simulink library "autolibshared"  (R2019b)
settings: Solver=ode45  StartTime=0.0  StopTime=10.0  RelTol=1e-3  EnableMultiTasking=on
undefined symbols (not defined in the file or in its folder): AccelCycle, aMode, DriveCycle, GearCycle, psi, x_o
libraries: autolibsharedcommon x20, $bdroot x7, autolibutils x2, autolibpowerinfoutils x1
(part 4 of 4)

== system autolibshared/Longitudinal Wheel/Wheel Module/Clutch/detectLockup/Friction Mode Logic ==
  note: Clutch Friction Mode Logic
  Tout : Inport
  Tfmaxs : Inport  Port=2
  locked_wout : Inport  Port=3
  Break Apart Detection : Subsystem
  Lockup Detection : Subsystem
  Lockup FSM : Subsystem
  Requisite Friction : Subsystem
  locked : Outport  InitialOutput=0  VectorParamsAs1DForOutWhenUnconnected=off
  wires:
  Tfmaxs/1 -> Break Apart Detection/1(Tfmaxs), Lockup Detection/2(Tfmaxs)
  Requisite Friction/1(Tf) -> Break Apart Detection/2(Tf)
  Break Apart Detection/1(unlock) -> Lockup FSM/2(unlock)
  Lockup Detection/1(lock) -> Lockup FSM/1(lock)
  Lockup FSM/1(locked) -> locked/1
  locked_wout/1 -> Requisite Friction/2(locked_w)
  Tout/1 -> Requisite Friction/1(Tout), Lockup Detection/1(Tout)

== system autolibshared/Longitudinal Wheel/Wheel Module/Clutch/detectSlip/Break Apart Detection ==
  Tfmaxs : Inport
  Tf : Inport  Port=2
  Abs : Abs  SaturateOnIntegerOverflow=on
  Relational Operator : RelationalOperator  OutDataTypeStr=boolean  RndMeth=Nearest  InputSameDT=on
  unlock : Outport  InitialOutput=0  VectorParamsAs1DForOutWhenUnconnected=off
  wires:
  Tf/1 -> Abs/1
  Relational Operator/1 -> unlock/1
  Abs/1 -> Relational Operator/1
  Tfmaxs/1 -> Relational Operator/2

== system autolibshared/Vehicle Body 3DOF Single Track/Cy/Cy table dual/For Each Subsystem ==
  alpha_f : Inport  Partition=on  PartitionDimension=1  PartitionWidth=1  PartitionOffset=0
  alpha_r : Inport  Port=2  Partition=on  PartitionDimension=1  PartitionWidth=1  PartitionOffset=0
  Cy_f(alpha_f) : Lookup_n-D  NumberOfTableDimensions=1  BreakpointsForDimension1=alpha_f_brk  Table=Cy_f_data  ExtrapMethod=Clip  InternalRulePriority=Speed  RndMeth=Simplest  InputSameDT=on
  Cy_r(alpha_r) : Lookup_n-D  NumberOfTableDimensions=1  BreakpointsForDimension1=alpha_r_brk  Table=Cy_r_data  ExtrapMethod=Clip  InternalRulePriority=Speed  RndMeth=Simplest  InputSameDT=on
  For Each : ForEach  DisableCoverage=on
  Cy_f : Outport  ConcatenationDimension=1  VectorParamsAs1DForOutWhenUnconnected=off
  Cy_r : Outport  Port=2  ConcatenationDimension=1  VectorParamsAs1DForOutWhenUnconnected=off
  wires:
  alpha_f/1 -> Cy_f(alpha_f)/1
  Cy_f(alpha_f)/1 -> Cy_f/1
  alpha_r/1 -> Cy_r(alpha_r)/1
  Cy_r(alpha_r)/1 -> Cy_r/1

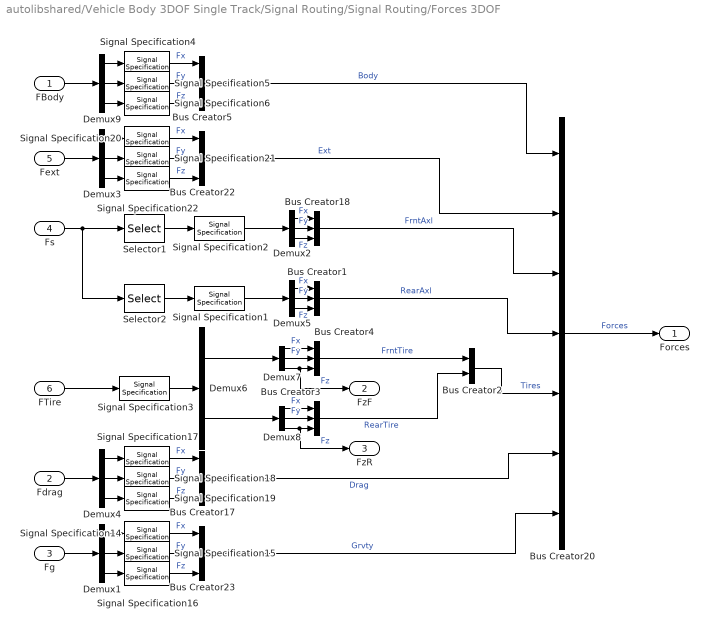
== system autolibshared/Vehicle Body 3DOF Single Track/Signal Routing/Signal Routing/Forces 3DOF ==
  FBody : Inport
  Fdrag : Inport  Port=2
  Fg : Inport  Port=3
  Fs : Inport  Port=4  Unit=N
  Fext : Inport  Port=5
  FTire : Inport  Port=6
  Bus Creator{1,3..5,17..18,22..23} (8 alike) : BusCreator  Inputs=3
  Bus Creator2 : BusCreator  Inputs=2
  Bus Creator20 : BusCreator  Inputs=7
  Demux{1..5,7..9} (8 alike) : Demux  Outputs=3
  Demux6 : Demux  Outputs=[3,3]
  Selector1 : Selector  IndexOptions=Index vector (dialog)  Indices=[1:3]  OutputSizes=1
  Selector2 : Selector  IndexOptions=Index vector (dialog)  Indices=[4:6]  OutputSizes=1
  Signal Specification{1..6,14..22} (15 alike) : SignalSpecification  Unit=N
  Forces : Outport  VectorParamsAs1DForOutWhenUnconnected=off
  FzF : Outport  Port=2  VectorParamsAs1DForOutWhenUnconnected=off
  FzR : Outport  Port=3  VectorParamsAs1DForOutWhenUnconnected=off
  wires:
  Signal Specification5/1 -> Bus Creator5/2  "Fy"
  Signal Specification4/1 -> Bus Creator5/1  "Fx"
  Signal Specification6/1 -> Bus Creator5/3  "Fz"
  FBody/1 -> Demux9/1
  Demux9/1 -> Signal Specification4/1
  Demux9/2 -> Signal Specification5/1
  Demux9/3 -> Signal Specification6/1
  Bus Creator5/1 -> Bus Creator20/1  "Body"
  Bus Creator17/1 -> Bus Creator20/6  "Drag"
  Bus Creator2/1 -> Bus Creator20/5  "Tires"
  Demux6/2 -> Demux8/1
  Demux6/1 -> Demux7/1
  Signal Specification3/1 -> Demux6/1
  FTire/1 -> Signal Specification3/1
  Selector2/1 -> Signal Specification1/1
  Signal Specification2/1 -> Demux2/1
  Signal Specification1/1 -> Demux5/1
  Fs/1 -> Selector2/1, Selector1/1
  Selector1/1 -> Signal Specification2/1
  Demux5/1 -> Bus Creator1/1  "Fx"
  Bus Creator4/1 -> Bus Creator2/1  "FrntTire"
  Bus Creator3/1 -> Bus Creator2/2  "RearTire"
  Demux7/1 -> Bus Creator4/1  "Fx"
  Demux7/2 -> Bus Creator4/2  "Fy"
  Demux7/3 -> Bus Creator4/3, FzF/1  "Fz"
  Demux8/3 -> Bus Creator3/3, FzR/1  "Fz"
  Demux8/2 -> Bus Creator3/2  "Fy"
  Demux8/1 -> Bus Creator3/1  "Fx"
  Demux5/2 -> Bus Creator1/2  "Fy"
  Demux5/3 -> Bus Creator1/3  "Fz"
  Demux2/3 -> Bus Creator18/3  "Fz"
  Demux2/2 -> Bus Creator18/2  "Fy"
  Demux2/1 -> Bus Creator18/1  "Fx"
  Bus Creator1/1 -> Bus Creator20/4  "RearAxl"
  Bus Creator18/1 -> Bus Creator20/3  "FrntAxl"
  Fdrag/1 -> Demux4/1
  Demux4/3 -> Signal Specification19/1
  Demux4/2 -> Signal Specification18/1
  Demux4/1 -> Signal Specification17/1
  Demux3/3 -> Signal Specification22/1
  Demux3/2 -> Signal Specification21/1
  Demux3/1 -> Signal Specification20/1
  Fext/1 -> Demux3/1
  Bus Creator22/1 -> Bus Creator20/2  "Ext"
  Signal Specification22/1 -> Bus Creator22/3  "Fz"
  Signal Specification20/1 -> Bus Creator22/1  "Fx"
  Signal Specification15/1 -> Bus Creator23/2  "Fy"
  Signal Specification21/1 -> Bus Creator22/2  "Fy"
  Signal Specification18/1 -> Bus Creator17/2  "Fy"
  Signal Specification17/1 -> Bus Creator17/1  "Fx"
  Signal Specification14/1 -> Bus Creator23/1  "Fx"
  Signal Specification19/1 -> Bus Creator17/3  "Fz"
  Signal Specification16/1 -> Bus Creator23/3  "Fz"
  Bus Creator20/1 -> Forces/1  "Forces"
  Bus Creator23/1 -> Bus Creator20/7  "Grvty"
  Demux1/2 -> Signal Specification15/1
  Demux1/3 -> Signal Specification16/1
  Fg/1 -> Demux1/1
  Demux1/1 -> Signal Specification14/1

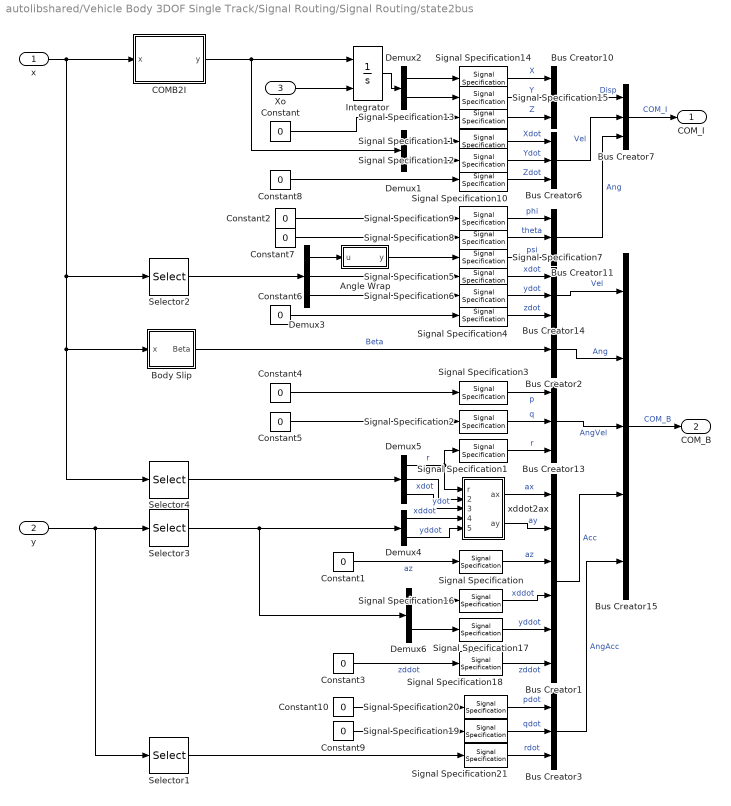
== system autolibshared/Vehicle Body 3DOF Single Track/Signal Routing/Signal Routing/state2bus ==
  x : Inport
  y : Inport  Port=2
  Xo : Inport  Port=3
  Angle Wrap : Subsystem  VariantControlMode=Label  Variant=on  VariantControl=Variant1  LabelModeActiveChoice=None
  Body Slip : Subsystem
  Bus Creator1 : BusCreator  Inputs=6
  Bus Creator{3,6..7,10..11,13..14} (7 alike) : BusCreator  Inputs=3
  Bus Creator15 : BusCreator  Inputs=5
  Bus Creator2 : BusCreator  Inputs=1
  COMB2I : MATLAB Function  TreatAsAtomicUnit=on
  Constant{,1..10} (11 alike) : Constant  Value=0
  Demux{1..2,4,6} (4 alike) : Demux  Outputs=2
  Demux3 : Demux  Outputs=3
  Demux5 : Demux  Outputs=3
  Integrator : Integrator  InitialConditionSource=external
  Selector1 : Selector  IndexOptions=Index vector (dialog)  Indices=[3]  OutputSizes=1
  Selector2 : Selector  IndexOptions=Index vector (dialog)  Indices=[3,1,2]  OutputSizes=1
  Selector3 : Selector  IndexOptions=Index vector (dialog)  Indices=[1,2]  OutputSizes=1
  Selector4 : Selector  IndexOptions=Index vector (dialog)  Indices=[4,1,2]  OutputSizes=1
  Signal Specification : SignalSpecification  Unit=gn
  Signal Specification1 : SignalSpecification  Unit=rad/s
  Signal Specification{4..6,10..12} (6 alike) : SignalSpecification  Unit=m/s
  Signal Specification13 : SignalSpecification  Unit=m
  Signal Specification14 : SignalSpecification  Unit=m
  Signal Specification15 : SignalSpecification  Unit=m
  Signal Specification16 : SignalSpecification  Unit=m/s^2
  Signal Specification17 : SignalSpecification  Unit=m/s^2
  Signal Specification18 : SignalSpecification  Unit=m/s^2
  Signal Specification19 : SignalSpecification  Unit=rad/s^2
  Signal Specification2 : SignalSpecification  Unit=rad/s
  Signal Specification20 : SignalSpecification  Unit=rad/s^2
  Signal Specification21 : SignalSpecification  Unit=rad/s^2
  Signal Specification3 : SignalSpecification  Unit=rad/s
  Signal Specification7 : SignalSpecification  Unit=rad
  Signal Specification8 : SignalSpecification  Unit=rad
  Signal Specification9 : SignalSpecification  Unit=rad
  xddot2ax : Subsystem
  COM_I : Outport  VectorParamsAs1DForOutWhenUnconnected=off
  COM_B : Outport  Port=2  VectorParamsAs1DForOutWhenUnconnected=off
  wires:
  Demux2/1 -> Signal Specification14/1
  Demux2/2 -> Signal Specification15/1
  Constant/1 -> Signal Specification13/1
  Demux1/1 -> Signal Specification11/1
  Demux1/2 -> Signal Specification12/1
  Constant2/1 -> Signal Specification9/1
  Constant7/1 -> Signal Specification8/1
  Demux3/1 -> Angle Wrap/1("u ")
  Demux3/3 -> Signal Specification6/1
  Demux3/2 -> Signal Specification5/1
  Constant6/1 -> Signal Specification4/1
  Constant4/1 -> Signal Specification3/1
  Constant5/1 -> Signal Specification2/1
  Signal Specification1/1 -> Bus Creator13/3  "r"
  xddot2ax/2(ay) -> Bus Creator1/2  "ay"
  xddot2ax/1(ax) -> Bus Creator1/1  "ax"
  Demux4/2 -> xddot2ax/5(yddot)  "yddot"
  Demux4/1 -> xddot2ax/4(xddot)  "xddot"
  Demux5/3 -> xddot2ax/3(ydot)  "ydot"
  Demux5/2 -> xddot2ax/2(xdot)  "xdot"
  Selector4/1 -> Demux5/1
  Demux5/1 -> xddot2ax/1(r), Signal Specification1/1  "r"
  x/1 -> Selector4/1, Body Slip/1(x), Selector2/1, COMB2I/1(x)
  Signal Specification10/1 -> Bus Creator6/3  "Zdot"
  Signal Specification4/1 -> Bus Creator14/3  "zdot"
  Signal Specification11/1 -> Bus Creator6/1  "Xdot"
  Signal Specification15/1 -> Bus Creator10/2  "Y"
  Bus Creator13/1 -> Bus Creator15/3  "AngVel"
  Signal Specification13/1 -> Bus Creator10/3  "Z"
  Signal Specification14/1 -> Bus Creator10/1  "X"
  Signal Specification9/1 -> Bus Creator11/1  "phi"
  Bus Creator7/1 -> COM_I/1  "COM_I"
  Signal Specification3/1 -> Bus Creator13/1  "p"
  Bus Creator14/1 -> Bus Creator15/1  "Vel"
  Bus Creator6/1 -> Bus Creator7/2  "Vel"
  Bus Creator10/1 -> Bus Creator7/1  "Disp"
  Signal Specification8/1 -> Bus Creator11/2  "theta"
  Selector2/1 -> Demux3/1
  Signal Specification12/1 -> Bus Creator6/2  "Ydot"
  Signal Specification2/1 -> Bus Creator13/2  "q"
  Bus Creator15/1 -> COM_B/1  "COM_B"
  Signal Specification5/1 -> Bus Creator14/1  "xdot"
  Bus Creator11/1 -> Bus Creator7/3  "Ang"
  Signal Specification6/1 -> Bus Creator14/2  "ydot"
  Integrator/1 -> Demux2/1
  COMB2I/1(y) -> Integrator/1, Demux1/1
  Signal Specification7/1 -> Bus Creator11/3  "psi"
  Signal Specification/1 -> Bus Creator1/3  "az"
  y/1 -> Selector1/1, Selector3/1
  Selector3/1 -> Demux4/1, Demux6/1
  Constant3/1 -> Signal Specification18/1  "zddot"
  Signal Specification18/1 -> Bus Creator1/6  "zddot"
  Signal Specification17/1 -> Bus Creator1/5  "yddot"
  Signal Specification16/1 -> Bus Creator1/4  "xddot"
  Constant1/1 -> Signal Specification/1  "az"
  Demux6/1 -> Signal Specification16/1
  Demux6/2 -> Signal Specification17/1
  Constant8/1 -> Signal Specification10/1
  Bus Creator1/1 -> Bus Creator15/4  "Acc"
  Bus Creator2/1 -> Bus Creator15/2  "Ang"
  Body Slip/1(Beta) -> Bus Creator2/1  "Beta"
  Xo/1 -> Integrator/2
  Signal Specification21/1 -> Bus Creator3/3  "rdot"
  Signal Specification19/1 -> Bus Creator3/2  "qdot"
  Signal Specification20/1 -> Bus Creator3/1  "pdot"
  Bus Creator3/1 -> Bus Creator15/5  "AngAcc"
  Constant9/1 -> Signal Specification19/1
  Constant10/1 -> Signal Specification20/1
  Selector1/1 -> Signal Specification21/1
  Angle Wrap/1(" y") -> Signal Specification7/1

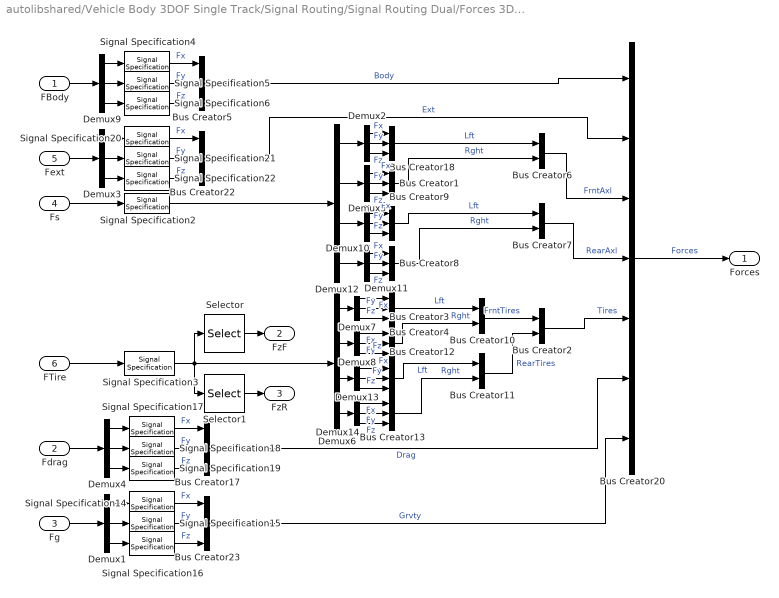
== system autolibshared/Vehicle Body 3DOF Single Track/Signal Routing/Signal Routing Dual/Forces 3DOF ==
  FBody : Inport
  Fdrag : Inport  Port=2
  Fg : Inport  Port=3
  Fs : Inport  Port=4  Unit=N
  Fext : Inport  Port=5
  FTire : Inport  Port=6
  Bus Creator{1,3..5,8..9,12..13,17..18,22..23} (12 alike) : BusCreator  Inputs=3
  Bus Creator{2,6..7,10..11} (5 alike) : BusCreator  Inputs=2
  Bus Creator20 : BusCreator  Inputs=7
  Demux{1..5,7..11,13..14} (12 alike) : Demux  Outputs=3
  Demux12 : Demux  Outputs=[3,3,3,3]
  Demux6 : Demux  Outputs=[3,3,3,3]
  Selector : Selector  InputPortWidth=12  IndexOptions=Index vector (dialog)  Indices=[3,6]  OutputSizes=1
  Selector1 : Selector  InputPortWidth=12  IndexOptions=Index vector (dialog)  Indices=[9,12]  OutputSizes=1
  Signal Specification{2..6,14..22} (14 alike) : SignalSpecification  Unit=N
  Forces : Outport  VectorParamsAs1DForOutWhenUnconnected=off
  FzF : Outport  Port=2  VectorParamsAs1DForOutWhenUnconnected=off
  FzR : Outport  Port=3  VectorParamsAs1DForOutWhenUnconnected=off
  wires:
  Selector1/1 -> FzR/1
  Selector/1 -> FzF/1
  Demux13/3 -> Bus Creator12/3  "Fz"
  Bus Creator13/1 -> Bus Creator11/2  "Rght"
  Demux14/1 -> Bus Creator13/1  "Fx"
  Demux14/2 -> Bus Creator13/2  "Fy"
  Demux14/3 -> Bus Creator13/3  "Fz"
  Demux6/4 -> Demux14/1
  Demux6/3 -> Demux13/1
  Demux13/2 -> Bus Creator12/2  "Fy"
  Demux13/1 -> Bus Creator12/1  "Fx"
  Signal Specification2/1 -> Demux12/1
  Bus Creator12/1 -> Bus Creator11/1  "Lft"
  Bus Creator3/1 -> Bus Creator10/2  "Rght"
  Bus Creator4/1 -> Bus Creator10/1  "Lft"
  Demux12/3 -> Demux10/1
  Demux12/4 -> Demux11/1
  Demux11/1 -> Bus Creator8/1  "Fx"
  Demux11/2 -> Bus Creator8/2  "Fy"
  Demux11/3 -> Bus Creator8/3  "Fz"
  Demux10/3 -> Bus Creator9/3  "Fz"
  Demux10/2 -> Bus Creator9/2  "Fy"
  Demux10/1 -> Bus Creator9/1  "Fx"
  Bus Creator9/1 -> Bus Creator7/1  "Lft"
  Bus Creator8/1 -> Bus Creator7/2  "Rght"
  Bus Creator1/1 -> Bus Creator6/2  "Rght"
  Bus Creator18/1 -> Bus Creator6/1  "Lft"
  Demux1/1 -> Signal Specification14/1
  Fg/1 -> Demux1/1
  Demux1/3 -> Signal Specification16/1
  Demux1/2 -> Signal Specification15/1
  Bus Creator23/1 -> Bus Creator20/7  "Grvty"
  Bus Creator20/1 -> Forces/1  "Forces"
  Signal Specification16/1 -> Bus Creator23/3  "Fz"
  Signal Specification19/1 -> Bus Creator17/3  "Fz"
  Signal Specification14/1 -> Bus Creator23/1  "Fx"
  Signal Specification17/1 -> Bus Creator17/1  "Fx"
  Signal Specification18/1 -> Bus Creator17/2  "Fy"
  Signal Specification21/1 -> Bus Creator22/2  "Fy"
  Signal Specification15/1 -> Bus Creator23/2  "Fy"
  Signal Specification20/1 -> Bus Creator22/1  "Fx"
  Signal Specification22/1 -> Bus Creator22/3  "Fz"
  Bus Creator22/1 -> Bus Creator20/2  "Ext"
  Fext/1 -> Demux3/1
  Demux3/1 -> Signal Specification20/1
  Demux3/2 -> Signal Specification21/1
  Demux3/3 -> Signal Specification22/1
  Demux4/1 -> Signal Specification17/1
  Demux4/2 -> Signal Specification18/1
  Demux4/3 -> Signal Specification19/1
  Fdrag/1 -> Demux4/1
  Bus Creator6/1 -> Bus Creator20/3  "FrntAxl"
  Bus Creator7/1 -> Bus Creator20/4  "RearAxl"
  Demux2/1 -> Bus Creator18/1  "Fx"
  Demux2/2 -> Bus Creator18/2  "Fy"
  Demux2/3 -> Bus Creator18/3  "Fz"
  Demux5/3 -> Bus Creator1/3  "Fz"
  Demux5/2 -> Bus Creator1/2  "Fy"
  Demux8/1 -> Bus Creator3/1  "Fx"
  Demux8/2 -> Bus Creator3/2  "Fy"
  Demux8/3 -> Bus Creator3/3  "Fz"
  Demux7/3 -> Bus Creator4/3  "Fz"
  Demux7/2 -> Bus Creator4/2  "Fy"
  Demux7/1 -> Bus Creator4/1  "Fx"
  Bus Creator11/1 -> Bus Creator2/2  "RearTires"
  Bus Creator10/1 -> Bus Creator2/1  "FrntTires"
  Demux5/1 -> Bus Creator1/1  "Fx"
  Fs/1 -> Signal Specification2/1
  Demux12/2 -> Demux5/1
  Demux12/1 -> Demux2/1
  FTire/1 -> Signal Specification3/1
  Signal Specification3/1 -> Demux6/1, Selector/1, Selector1/1
  Demux6/1 -> Demux7/1
  Demux6/2 -> Demux8/1
  Bus Creator2/1 -> Bus Creator20/5  "Tires"
  Bus Creator17/1 -> Bus Creator20/6  "Drag"
  Bus Creator5/1 -> Bus Creator20/1  "Body"
  Demux9/3 -> Signal Specification6/1
  Demux9/2 -> Signal Specification5/1
  Demux9/1 -> Signal Specification4/1
  FBody/1 -> Demux9/1
  Signal Specification6/1 -> Bus Creator5/3  "Fz"
  Signal Specification4/1 -> Bus Creator5/1  "Fx"
  Signal Specification5/1 -> Bus Creator5/2  "Fy"

== system autolibshared/Vehicle Body 3DOF Single Track/Signal Routing/Signal Routing Dual/Lateral 3DOF ==
  InertCg : Inport
  BdyFrmCg : Inport  Port=2
  Forces : Inport  Port=3
  Power : Inport  Port=4
  Moments : Inport  Port=5
  WhlAngF : Inport  Port=6
  WhlAngR : Inport  Port=7
  Bus Creator1 : BusCreator  Inputs=7
  Bus Creator2 : BusCreator  Inputs=4
  Bus Creator{3..4,7..8} (4 alike) : BusCreator  Inputs=2
  Bus Creator5 : BusCreator  Inputs=3
  Bus Creator6 : BusCreator  Inputs=3
  Bus Selector : BusSelector  OutputSignals=Pwr,PwrInfo
  Demux : Demux  Outputs=2
  Demux1 : Demux  Outputs=2
  Hard Point Coordinate Transform Front Left : Subsystem
  Hard Point Coordinate Transform Front Right : Subsystem
  Hard Point Coordinate Transform Geometric : Subsystem
  Hard Point Coordinate Transform Rear Left : Subsystem
  Hard Point Coordinate Transform Rear Right : Subsystem
  InertFrm : Outport  VectorParamsAs1DForOutWhenUnconnected=off
  BdyFrm : Outport  Port=2  VectorParamsAs1DForOutWhenUnconnected=off
  PwrInfo : Outport  Port=3  VectorParamsAs1DForOutWhenUnconnected=off
  wires:
  Bus Creator6/1 -> Bus Creator1/5  "RearAxl"
  Hard Point Coordinate Transform Front Left/2(Body) -> Bus Creator5/1  "Lft"
  Hard Point Coordinate Transform Front Right/2(Body) -> Bus Creator5/2  "Rght"
  Hard Point Coordinate Transform Rear Left/2(Body) -> Bus Creator6/1  "Lft"
  Hard Point Coordinate Transform Rear Right/2(Body) -> Bus Creator6/2  "Rght"
  Hard Point Coordinate Transform Rear Right/1(Inert) -> Bus Creator4/2  "Rght"
  Hard Point Coordinate Transform Rear Left/1(Inert) -> Bus Creator4/1  "Lft"
  Hard Point Coordinate Transform Front Right/1(Inert) -> Bus Creator3/2  "Rght"
  Hard Point Coordinate Transform Front Left/1(Inert) -> Bus Creator3/1  "Lft"
  Moments/1 -> Bus Creator1/3  "Moments"
  Bus Creator5/1 -> Bus Creator1/4  "FrntAxl"
  InertCg/1 -> Hard Point Coordinate Transform Front Left/1(InertFrmCg), Bus Creator2/1, Hard Point Coordinate Transform Front Right/1(InertFrmCg), Hard Point Coordinate Transform Geometric/1(InertFrmCg), Hard Point Coordinate Transform Rear Right/1(InertFrmCg), Hard Point Coordinate Transform Rear Left/1(InertFrmCg)  "Cg"
  Bus Creator4/1 -> Bus Creator2/3  "RearAxl"
  Bus Creator2/1 -> InertFrm/1  "InertFrm"
  Bus Creator1/1 -> BdyFrm/1  "BdyFrm"
  Bus Creator3/1 -> Bus Creator2/2  "FrntAxl"
  BdyFrmCg/1 -> Hard Point Coordinate Transform Geometric/2(BdyFrmCg), Bus Creator1/1, Hard Point Coordinate Transform Rear Right/2(BdyFrmCg), Hard Point Coordinate Transform Rear Left/2(BdyFrmCg), Hard Point Coordinate Transform Front Right/2(BdyFrmCg), Hard Point Coordinate Transform Front Left/2(BdyFrmCg)  "Cg"
  Forces/1 -> Bus Creator1/2  "Forces"
  Hard Point Coordinate Transform Geometric/2(Body) -> Bus Creator1/7  "Geom"
  Hard Point Coordinate Transform Geometric/1(Inert) -> Bus Creator2/4  "Geom"
  WhlAngF/1 -> Demux/1  "WhlAngF"
  WhlAngR/1 -> Demux1/1  "WhlAngR"
  Bus Creator7/1 -> Bus Creator6/3  "Steer"
  Bus Creator8/1 -> Bus Creator5/3  "Steer"
  Demux/1 -> Bus Creator8/1  "WhlAngFL"
  Demux/2 -> Bus Creator8/2  "WhlAngFR"
  Demux1/1 -> Bus Creator7/1  "WhlAngRL"
  Demux1/2 -> Bus Creator7/2  "WhlAngRR"
  Bus Selector/2 -> PwrInfo/1  "<PwrInfo>"
  Bus Selector/1 -> Bus Creator1/6  "<Pwr>"
  Power/1 -> Bus Selector/1  "Pwr"

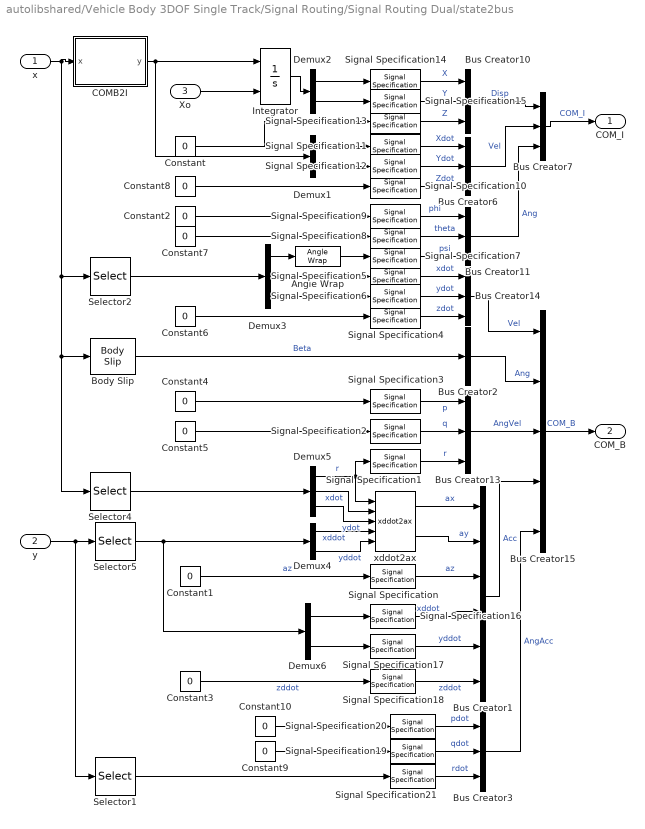
== system autolibshared/Vehicle Body 3DOF Single Track/Signal Routing/Signal Routing Dual/state2bus ==
  x : Inport
  y : Inport  Port=2
  Xo : Inport  Port=3
  Angle Wrap : $bdroot/Vehicle Body 3DOF Single Track/Signal Routing/Signal Routing/state2bus/Angle Wrap  SystemSampleTime=-1  VariantControl=Variant1  LabelModeActiveChoice=None  Latency=0  AutoFrameSizeCalculation=off
  Body Slip : $bdroot/Vehicle Body 3DOF Single Track/Signal Routing/Signal Routing/state2bus/Body Slip  SystemSampleTime=-1  Latency=0  AutoFrameSizeCalculation=off
  Bus Creator1 : BusCreator  Inputs=6
  Bus Creator{3,6..7,10..11,13..14} (7 alike) : BusCreator  Inputs=3
  Bus Creator15 : BusCreator  Inputs=5
  Bus Creator2 : BusCreator  Inputs=1
  COMB2I : MATLAB Function  TreatAsAtomicUnit=on
  Constant{,1..10} (11 alike) : Constant  Value=0
  Demux{1..2,4,6} (4 alike) : Demux  Outputs=2
  Demux3 : Demux  Outputs=3
  Demux5 : Demux  Outputs=3
  Integrator : Integrator  InitialConditionSource=external
  Selector1 : Selector  IndexOptions=Index vector (dialog)  Indices=[3]  OutputSizes=1
  Selector2 : Selector  IndexOptions=Index vector (dialog)  Indices=[3,1,2]  OutputSizes=1
  Selector4 : Selector  IndexOptions=Index vector (dialog)  Indices=[4,1,2]  OutputSizes=1
  Selector5 : Selector  IndexOptions=Index vector (dialog)  Indices=[1,2]  OutputSizes=1
  Signal Specification : SignalSpecification  Unit=gn
  Signal Specification1 : SignalSpecification  Unit=rad/s
  Signal Specification{4..6,10..12} (6 alike) : SignalSpecification  Unit=m/s
  Signal Specification13 : SignalSpecification  Unit=m
  Signal Specification14 : SignalSpecification  Unit=m
  Signal Specification15 : SignalSpecification  Unit=m
  Signal Specification16 : SignalSpecification  Unit=m/s^2
  Signal Specification17 : SignalSpecification  Unit=m/s^2
  Signal Specification18 : SignalSpecification  Unit=m/s^2
  Signal Specification19 : SignalSpecification  Unit=rad/s^2
  Signal Specification2 : SignalSpecification  Unit=rad/s
  Signal Specification20 : SignalSpecification  Unit=rad/s^2
  Signal Specification21 : SignalSpecification  Unit=rad/s^2
  Signal Specification3 : SignalSpecification  Unit=rad/s
  Signal Specification7 : SignalSpecification  Unit=rad
  Signal Specification8 : SignalSpecification  Unit=rad
  Signal Specification9 : SignalSpecification  Unit=rad
  xddot2ax : $bdroot/Vehicle Body 3DOF Single Track/Signal Routing/Signal Routing/state2bus/xddot2ax  SystemSampleTime=-1  Latency=0  AutoFrameSizeCalculation=off
  COM_I : Outport  VectorParamsAs1DForOutWhenUnconnected=off
  COM_B : Outport  Port=2  VectorParamsAs1DForOutWhenUnconnected=off
  wires:
  Signal Specification7/1 -> Bus Creator11/3  "psi"
  COMB2I/1(y) -> Demux1/1, Integrator/1
  Integrator/1 -> Demux2/1
  Signal Specification6/1 -> Bus Creator14/2  "ydot"
  Bus Creator11/1 -> Bus Creator7/3  "Ang"
  Signal Specification5/1 -> Bus Creator14/1  "xdot"
  Bus Creator15/1 -> COM_B/1  "COM_B"
  Signal Specification2/1 -> Bus Creator13/2  "q"
  Signal Specification12/1 -> Bus Creator6/2  "Ydot"
  Selector2/1 -> Demux3/1
  Signal Specification8/1 -> Bus Creator11/2  "theta"
  Bus Creator10/1 -> Bus Creator7/1  "Disp"
  Bus Creator6/1 -> Bus Creator7/2  "Vel"
  Bus Creator14/1 -> Bus Creator15/1  "Vel"
  Signal Specification3/1 -> Bus Creator13/1  "p"
  Bus Creator7/1 -> COM_I/1  "COM_I"
  Signal Specification9/1 -> Bus Creator11/1  "phi"
  Signal Specification14/1 -> Bus Creator10/1  "X"
  Signal Specification13/1 -> Bus Creator10/3  "Z"
  Bus Creator13/1 -> Bus Creator15/3  "AngVel"
  Signal Specification15/1 -> Bus Creator10/2  "Y"
  Signal Specification11/1 -> Bus Creator6/1  "Xdot"
  Signal Specification4/1 -> Bus Creator14/3  "zdot"
  Signal Specification10/1 -> Bus Creator6/3  "Zdot"
  x/1 -> COMB2I/1(x), Selector2/1, Body Slip/1, Selector4/1
  Signal Specification1/1 -> Bus Creator13/3  "r"
  Constant5/1 -> Signal Specification2/1
  Constant4/1 -> Signal Specification3/1
  Constant6/1 -> Signal Specification4/1
  Demux3/2 -> Signal Specification5/1
  Demux3/3 -> Signal Specification6/1
  Demux3/1 -> Angle Wrap/1
  Constant7/1 -> Signal Specification8/1
  Constant2/1 -> Signal Specification9/1
  Constant8/1 -> Signal Specification10/1
  Demux1/2 -> Signal Specification12/1
  Demux1/1 -> Signal Specification11/1
  Constant/1 -> Signal Specification13/1
  Demux2/2 -> Signal Specification15/1
  Demux2/1 -> Signal Specification14/1
  y/1 -> Selector1/1, Selector5/1
  Demux5/2 -> xddot2ax/2  "xdot"
  Demux4/1 -> xddot2ax/4  "xddot"
  Selector4/1 -> Demux5/1
  Constant1/1 -> Signal Specification/1  "az"
  Demux5/3 -> xddot2ax/3  "ydot"
  Signal Specification/1 -> Bus Creator1/3  "az"
  Constant3/1 -> Signal Specification18/1  "zddot"
  Demux4/2 -> xddot2ax/5  "yddot"
  Selector5/1 -> Demux4/1, Demux6/1
  xddot2ax/2 -> Bus Creator1/2  "ay"
  Demux5/1 -> Signal Specification1/1, xddot2ax/1  "r"
  xddot2ax/1 -> Bus Creator1/1  "ax"
  Bus Creator1/1 -> Bus Creator15/4  "Acc"
  Signal Specification17/1 -> Bus Creator1/5  "yddot"
  Signal Specification18/1 -> Bus Creator1/6  "zddot"
  Signal Specification16/1 -> Bus Creator1/4  "xddot"
  Demux6/1 -> Signal Specification16/1
  Demux6/2 -> Signal Specification17/1
  Body Slip/1 -> Bus Creator2/1  "Beta"
  Bus Creator2/1 -> Bus Creator15/2  "Ang"
  Xo/1 -> Integrator/2
  Signal Specification21/1 -> Bus Creator3/3  "rdot"
  Signal Specification19/1 -> Bus Creator3/2  "qdot"
  Selector1/1 -> Signal Specification21/1
  Signal Specification20/1 -> Bus Creator3/1  "pdot"
  Constant9/1 -> Signal Specification19/1
  Bus Creator3/1 -> Bus Creator15/5  "AngAcc"
  Constant10/1 -> Signal Specification20/1
  Angle Wrap/1 -> Signal Specification7/1

== system autolibshared/Vehicle Body 3DOF Single Track/sigma/sigma/relaxation front ==
  alpha : Inport
  V : Inport  Port=2
  sigma : Inport  Port=3
  Product1 : Product  Inputs=**/  SaturateOnIntegerOverflow=on  RndMeth=Zero  InputSameDT=on  OutDataTypeStr=Inherit: Same as first input
  Sum : Sum  Inputs=-+|  SaturateOnIntegerOverflow=on  InputSameDT=on  OutDataTypeStr=Inherit: Same as first input
  lateral : Integrator
  alpha_sig : Outport  VectorParamsAs1DForOutWhenUnconnected=off
  wires:
  alpha/1 -> Sum/2
  V/1 -> Product1/2
  Product1/1 -> lateral/1
  Sum/1 -> Product1/1
  sigma/1 -> Product1/3
  lateral/1 -> Sum/1, alpha_sig/1

== system autolibshared/Vehicle Body 3DOF Single Track/sigma/sigma/relaxation rear ==
  alpha : Inport
  V : Inport  Port=2
  sigma : Inport  Port=3
  Product1 : Product  Inputs=**/  SaturateOnIntegerOverflow=on  RndMeth=Zero  InputSameDT=on  OutDataTypeStr=Inherit: Same as first input
  Sum : Sum  Inputs=-+|  SaturateOnIntegerOverflow=on  InputSameDT=on  OutDataTypeStr=Inherit: Same as first input
  lateral : Integrator
  alpha_sig : Outport  VectorParamsAs1DForOutWhenUnconnected=off
  wires:
  lateral/1 -> Sum/1, alpha_sig/1
  sigma/1 -> Product1/3
  Sum/1 -> Product1/1
  Product1/1 -> lateral/1
  V/1 -> Product1/2
  alpha/1 -> Sum/2

== system autolibshared/Vehicle Body 3DOF Single Track/sigma/sigma dual/relaxation ==
  alpha : Inport
  V : Inport  Port=2
  sigma : Inport  Port=3
  Product1 : Product  Inputs=**/  SaturateOnIntegerOverflow=on  RndMeth=Zero  InputSameDT=on  OutDataTypeStr=Inherit: Same as first input
  Sum : Sum  Inputs=-+|  SaturateOnIntegerOverflow=on  InputSameDT=on  OutDataTypeStr=Inherit: Same as first input
  lateral : Integrator
  alpha_sig : Outport  VectorParamsAs1DForOutWhenUnconnected=off
  wires:
  lateral/1 -> alpha_sig/1, Sum/1
  sigma/1 -> Product1/3
  Sum/1 -> Product1/1
  Product1/1 -> lateral/1
  V/1 -> Product1/2
  alpha/1 -> Sum/2

== system autolibshared/Longitudinal Wheel/Wheel Module/Brakes/Drum Brake/Drum Brake ==
  Brake Pressure : Inport
  Wheel angular velocity : Inport  Port=2
  Brake Actuator Bore : Constant  Value=drum_abore
  Disallow Negative Brake Torque : Saturate  UpperLimit=inf  LowerLimit=eps  ZeroCross=off
  Drum Brake Torque Calculation : MATLAB Function  TreatAsAtomicUnit=on
  Drum internal radius : Constant  Value=drum_r
  Kinetic friction coefficient : Constant  Value=mu_kinetic
  Shoe pin center to force application point distance : Constant  Value=drum_c
  Shoe pin to drum center distance : Constant  Value=drum_a
  Shoe pin to pad end angle : Constant  Value=drum_theta2
  Shoe pin to pad start angle : Constant  Value=drum_theta1
  Terminator : Terminator
  Brake Torque : Outport  VectorParamsAs1DForOutWhenUnconnected=off
  wires:
  Disallow Negative Brake Torque/1 -> Brake Torque/1
  Brake Actuator Bore/1 -> Drum Brake Torque Calculation/2(Ba)
  Wheel angular velocity/1 -> Terminator/1
  Shoe pin to drum center distance/1 -> Drum Brake Torque Calculation/4(a)
  Shoe pin center to force application point distance/1 -> Drum Brake Torque Calculation/5(c)
  Drum internal radius/1 -> Drum Brake Torque Calculation/6(r)
  Drum Brake Torque Calculation/1(T) -> Disallow Negative Brake Torque/1
  Kinetic friction coefficient/1 -> Drum Brake Torque Calculation/3(mu)
  Shoe pin to pad start angle/1 -> Drum Brake Torque Calculation/7(theta1)
  Shoe pin to pad end angle/1 -> Drum Brake Torque Calculation/8(theta2)
  Brake Pressure/1 -> Drum Brake Torque Calculation/1(P)

== system autolibshared/Longitudinal Wheel/Wheel Module/Clutch/detectLockup/Friction Mode Logic/Break Apart Detection ==
  Tfmaxs : Inport
  Tf : Inport  Port=2
  Abs : Abs  ZeroCross=off  SaturateOnIntegerOverflow=on
  Relational Operator : RelationalOperator  OutDataTypeStr=boolean  ZeroCross=off  RndMeth=Nearest  InputSameDT=on
  unlock : Outport  InitialOutput=0  VectorParamsAs1DForOutWhenUnconnected=off
  wires:
  Tf/1 -> Abs/1
  Relational Operator/1 -> unlock/1
  Abs/1 -> Relational Operator/1
  Tfmaxs/1 -> Relational Operator/2

== system autolibshared/Longitudinal Wheel/Wheel Module/Clutch/detectLockup/Friction Mode Logic/Lockup Detection ==
  Tout : Inport
  Tfmaxs : Inport  Port=2
  Friction Calc : Subsystem
  Required Friction for Lockup : Subsystem
  lock : Outport  InitialOutput=0  VectorParamsAs1DForOutWhenUnconnected=off
  wires:
  Tout/1 -> Friction Calc/1(Tout)
  Friction Calc/1(Friction Torque) -> Required Friction for Lockup/1(Friction Torque)
  Tfmaxs/1 -> Required Friction for Lockup/2(Max Friction Torque)
  Required Friction for Lockup/1(okay) -> lock/1

== system autolibshared/Longitudinal Wheel/Wheel Module/Clutch/detectLockup/Friction Mode Logic/Lockup FSM ==
  lock : Inport
  unlock : Inport  Port=2
  Combinatorial Logic : CombinatorialLogic  TruthTable=[0;1;0;0;1;1;1;0]
  Mux : Mux  Inputs=3
  Unit Delay : UnitDelay  SampleTime=-1  HasFrameUpgradeWarning=on
  locked : Outport  InitialOutput=0  VectorParamsAs1DForOutWhenUnconnected=off
  wires:
  Combinatorial Logic/1 -> Unit Delay/1, locked/1
  unlock/1 -> Mux/2
  lock/1 -> Mux/1
  Mux/1 -> Combinatorial Logic/1
  Unit Delay/1 -> Mux/3

== system autolibshared/Longitudinal Wheel/Wheel Module/Clutch/detectLockup/Friction Mode Logic/Requisite Friction ==
  Tout : Inport
  locked_w : Inport  Port=2
  Output Damping : Gain  Gain=1e-3  SaturateOnIntegerOverflow=on  OutDataTypeStr=Inherit: Same as input  ParamDataTypeStr=Inherit: Same as input
  Sum1 : Sum  Inputs=|++  SaturateOnIntegerOverflow=on  InputSameDT=on  OutDataTypeStr=Inherit: Same as first input
  Sum2 : Sum  Inputs=|--  SaturateOnIntegerOverflow=on  InputSameDT=on  OutDataTypeStr=Inherit: Same as first input
  Tf : Outport  InitialOutput=0  VectorParamsAs1DForOutWhenUnconnected=off
  wires:
  Sum1/1 -> Tf/1
  Sum2/1 -> Sum1/1
  Tout/1 -> Sum2/1
  locked_w/1 -> Output Damping/1
  Output Damping/1 -> Sum2/2, Sum1/2

== system autolibshared/Vehicle Body 3DOF Single Track/Signal Routing/Signal Routing/state2bus/Angle Wrap ==
  "u " : Inport
  None : Subsystem  VariantControl=None
  Wrap : autolibutils/Wrap  VariantControl=Wrap  aMode=aMode
      settings: SourceProductName=Powertrain Blockset  SourceProductBaseCode=PW
  " y" : Outport  VectorParamsAs1DForOutWhenUnconnected=off

== system autolibshared/Vehicle Body 3DOF Single Track/Signal Routing/Signal Routing/state2bus/Body Slip ==
  x : Inport
  Demux7 : Demux  Outputs=2
  Divide : Product  Inputs=*/
  Selector1 : Selector  IndexOptions=Index vector (dialog)  Indices=[2,1]  OutputSizes=1
  Signal Specification9 : SignalSpecification  Unit=rad
  Trigonometric Function : Trigonometry  Operator=atan  OutputSignalType=real
  div0protect - abs poly : autolibutils/div0protect - abs poly  thresh=xdot_tol  aMode=aMode
      settings: SourceProductName=Powertrain Blockset  SourceProductBaseCode=PW
  Beta : Outport  VectorParamsAs1DForOutWhenUnconnected=off
  wires:
  Demux7/2 -> div0protect - abs poly/1
  div0protect - abs poly/1 -> Divide/2
  Demux7/1 -> Divide/1
  x/1 -> Selector1/1
  Selector1/1 -> Demux7/1
  Trigonometric Function/1 -> Signal Specification9/1  "Beta"
  Divide/1 -> Trigonometric Function/1
  Signal Specification9/1 -> Beta/1

== system autolibshared/Vehicle Body 3DOF Single Track/Signal Routing/Signal Routing/state2bus/xddot2ax ==
  r : Inport
  xdot : Inport  Port=2
  ydot : Inport  Port=3
  xddot : Inport  Port=4
  yddot : Inport  Port=5
  Divide : Product  Inputs=**
  Divide1 : Product  Inputs=**
  Sum of Elements : Sum
  Sum of Elements1 : Sum  Inputs=-+
  m^22gn : Subsystem
  ax : Outport  Unit=gn  VectorParamsAs1DForOutWhenUnconnected=off
  ay : Outport  Port=2  Unit=gn  VectorParamsAs1DForOutWhenUnconnected=off
  wires:
  m^22gn/1(ay_g) -> ay/1
  m^22gn/2(ax_g) -> ax/1
  Sum of Elements1/1 -> m^22gn/2(ax)  "ax"
  Sum of Elements/1 -> m^22gn/1(ay)  "ay"
  yddot/1 -> Sum of Elements/1
  Divide1/1 -> Sum of Elements1/1
  Divide/1 -> Sum of Elements/2
  r/1 -> Divide1/1, Divide/2
  ydot/1 -> Divide1/2
  xdot/1 -> Divide/1
  xddot/1 -> Sum of Elements1/2

== system autolibshared/Vehicle Body 3DOF Single Track/Signal Routing/Signal Routing Dual/Lateral 3DOF/Hard Point Coordinate Transform Front Left ==
  InertFrmCg : Inport
  BdyFrmCg : Inport  Port=2
  Gain : Gain  Gain=-1/2
  Hard Point Coordinate Transform External Displacement : autolibsharedcommon/Hard Point Coordinate Transform External Displacement  aMode=aMode
      settings: SourceProductName=Powertrain Blockset  SourceProductBaseCode=PW
  Selector : Selector  InputPortWidth=2  IndexOptions=Index vector (dialog)  Indices=[1]  OutputSizes=1
  Subtract : Sum  Inputs=+-
  Vector Concatenate : Concatenate  NumInputs=3
  a : Constant  Value=a
  d : Constant  Value=d
  h : Constant  Value=h
  w : Constant  Value=w
  Inert : Outport  VectorParamsAs1DForOutWhenUnconnected=off
  Body : Outport  Port=2  VectorParamsAs1DForOutWhenUnconnected=off
  wires:
  Selector/1 -> Gain/1
  Hard Point Coordinate Transform External Displacement/1 -> Inert/1
  BdyFrmCg/1 -> Hard Point Coordinate Transform External Displacement/2
  h/1 -> Vector Concatenate/3
  Vector Concatenate/1 -> Hard Point Coordinate Transform External Displacement/3
  Hard Point Coordinate Transform External Displacement/2 -> Body/1
  a/1 -> Vector Concatenate/1
  Gain/1 -> Subtract/1
  w/1 -> Selector/1
  InertFrmCg/1 -> Hard Point Coordinate Transform External Displacement/1
  d/1 -> Subtract/2
  Subtract/1 -> Vector Concatenate/2

== system autolibshared/Vehicle Body 3DOF Single Track/Signal Routing/Signal Routing Dual/Lateral 3DOF/Hard Point Coordinate Transform Front Right ==
  InertFrmCg : Inport
  BdyFrmCg : Inport  Port=2
  Gain : Gain  Gain=1/2
  Hard Point Coordinate Transform External Displacement : autolibsharedcommon/Hard Point Coordinate Transform External Displacement  aMode=aMode
      settings: SourceProductName=Powertrain Blockset  SourceProductBaseCode=PW
  Selector : Selector  InputPortWidth=2  IndexOptions=Index vector (dialog)  Indices=[1]  OutputSizes=1
  Subtract : Sum  Inputs=+-
  Vector Concatenate : Concatenate  NumInputs=3
  a : Constant  Value=a
  d : Constant  Value=d
  h : Constant  Value=h
  w : Constant  Value=w
  Inert : Outport  VectorParamsAs1DForOutWhenUnconnected=off
  Body : Outport  Port=2  VectorParamsAs1DForOutWhenUnconnected=off
  wires:
  InertFrmCg/1 -> Hard Point Coordinate Transform External Displacement/1
  Hard Point Coordinate Transform External Displacement/2 -> Body/1
  Vector Concatenate/1 -> Hard Point Coordinate Transform External Displacement/3
  BdyFrmCg/1 -> Hard Point Coordinate Transform External Displacement/2
  Hard Point Coordinate Transform External Displacement/1 -> Inert/1
  Gain/1 -> Subtract/1
  d/1 -> Subtract/2
  w/1 -> Selector/1
  h/1 -> Vector Concatenate/3
  Selector/1 -> Gain/1
  a/1 -> Vector Concatenate/1
  Subtract/1 -> Vector Concatenate/2

== system autolibshared/Vehicle Body 3DOF Single Track/Signal Routing/Signal Routing Dual/Lateral 3DOF/Hard Point Coordinate Transform Geometric ==
  InertFrmCg : Inport
  BdyFrmCg : Inport  Port=2
  Hard Point Coordinate Transform External Displacement Beta : autolibsharedcommon/Hard Point Coordinate Transform External Displacement Beta  xdot_tol=xdot_tol  aMode=aMode
      settings: SourceProductName=Powertrain Blockset  SourceProductBaseCode=PW
  Vector Concatenate : Concatenate  NumInputs=3
  latOff : Constant  Value=latOff
  longOff : Constant  Value=longOff
  vertOff : Constant  Value=vertOff
  Inert : Outport  VectorParamsAs1DForOutWhenUnconnected=off
  Body : Outport  Port=2  VectorParamsAs1DForOutWhenUnconnected=off
  wires:
  latOff/1 -> Vector Concatenate/2
  longOff/1 -> Vector Concatenate/1
  vertOff/1 -> Vector Concatenate/3
  Hard Point Coordinate Transform External Displacement Beta/1 -> Inert/1
  BdyFrmCg/1 -> Hard Point Coordinate Transform External Displacement Beta/2
  Vector Concatenate/1 -> Hard Point Coordinate Transform External Displacement Beta/3
  Hard Point Coordinate Transform External Displacement Beta/2 -> Body/1
  InertFrmCg/1 -> Hard Point Coordinate Transform External Displacement Beta/1

== system autolibshared/Vehicle Body 3DOF Single Track/Signal Routing/Signal Routing Dual/Lateral 3DOF/Hard Point Coordinate Transform Rear Left ==
  InertFrmCg : Inport
  BdyFrmCg : Inport  Port=2
  Gain : Gain  Gain=-1/2
  Hard Point Coordinate Transform External Displacement : autolibsharedcommon/Hard Point Coordinate Transform External Displacement  aMode=aMode
      settings: SourceProductName=Powertrain Blockset  SourceProductBaseCode=PW
  Selector : Selector  InputPortWidth=2  IndexOptions=Index vector (dialog)  Indices=[2]  OutputSizes=1
  Subtract : Sum  Inputs=+-
  Vector Concatenate : Concatenate  NumInputs=3
  b : Constant  Value=-b
  d : Constant  Value=d
  h : Constant  Value=h
  w : Constant  Value=w
  Inert : Outport  VectorParamsAs1DForOutWhenUnconnected=off
  Body : Outport  Port=2  VectorParamsAs1DForOutWhenUnconnected=off
  wires:
  Hard Point Coordinate Transform External Displacement/1 -> Inert/1
  BdyFrmCg/1 -> Hard Point Coordinate Transform External Displacement/2
  Vector Concatenate/1 -> Hard Point Coordinate Transform External Displacement/3
  Hard Point Coordinate Transform External Displacement/2 -> Body/1
  InertFrmCg/1 -> Hard Point Coordinate Transform External Displacement/1
  h/1 -> Vector Concatenate/3
  b/1 -> Vector Concatenate/1
  Selector/1 -> Gain/1
  d/1 -> Subtract/2
  w/1 -> Selector/1
  Subtract/1 -> Vector Concatenate/2
  Gain/1 -> Subtract/1

== system autolibshared/Vehicle Body 3DOF Single Track/Signal Routing/Signal Routing Dual/Lateral 3DOF/Hard Point Coordinate Transform Rear Right ==
  InertFrmCg : Inport
  BdyFrmCg : Inport  Port=2
  Gain : Gain  Gain=1/2
  Hard Point Coordinate Transform External Displacement : autolibsharedcommon/Hard Point Coordinate Transform External Displacement  aMode=aMode
      settings: SourceProductName=Powertrain Blockset  SourceProductBaseCode=PW
  Selector : Selector  InputPortWidth=2  IndexOptions=Index vector (dialog)  Indices=[2]  OutputSizes=1
  Subtract : Sum  Inputs=+-
  Vector Concatenate : Concatenate  NumInputs=3
  b : Constant  Value=-b
  d : Constant  Value=d
  h : Constant  Value=h
  w : Constant  Value=w
  Inert : Outport  VectorParamsAs1DForOutWhenUnconnected=off
  Body : Outport  Port=2  VectorParamsAs1DForOutWhenUnconnected=off
  wires:
  InertFrmCg/1 -> Hard Point Coordinate Transform External Displacement/1
  Hard Point Coordinate Transform External Displacement/2 -> Body/1
  Vector Concatenate/1 -> Hard Point Coordinate Transform External Displacement/3
  BdyFrmCg/1 -> Hard Point Coordinate Transform External Displacement/2
  Hard Point Coordinate Transform External Displacement/1 -> Inert/1
  h/1 -> Vector Concatenate/3
  b/1 -> Vector Concatenate/1
  Selector/1 -> Gain/1
  d/1 -> Subtract/2
  w/1 -> Selector/1
  Subtract/1 -> Vector Concatenate/2
  Gain/1 -> Subtract/1

== system autolibshared/Longitudinal Wheel/Wheel Module/Clutch/detectLockup/Friction Mode Logic/Lockup Detection/Friction Calc ==
  Tout : Inport
  Unary Minus : UnaryMinus
  Friction Torque : Outport  InitialOutput=0  VectorParamsAs1DForOutWhenUnconnected=off
  wires:
  Unary Minus/1 -> Friction Torque/1
  Tout/1 -> Unary Minus/1

== system autolibshared/Longitudinal Wheel/Wheel Module/Clutch/detectLockup/Friction Mode Logic/Lockup Detection/Required Friction for Lockup ==
  Friction Torque : Inport
  Max Friction Torque : Inport  Port=2
  Abs : Abs  ZeroCross=off  SaturateOnIntegerOverflow=on
  Relational Operator : RelationalOperator  Operator=<=  OutDataTypeStr=boolean  ZeroCross=off  RndMeth=Nearest  InputSameDT=on
  okay : Outport  InitialOutput=0  VectorParamsAs1DForOutWhenUnconnected=off
  wires:
  Friction Torque/1 -> Abs/1
  Relational Operator/1 -> okay/1
  Abs/1 -> Relational Operator/1
  Max Friction Torque/1 -> Relational Operator/2

== system autolibshared/Vehicle Body 3DOF Single Track/Signal Routing/Signal Routing/state2bus/Angle Wrap/None ==
  u : Inport
  y : Outport  VectorParamsAs1DForOutWhenUnconnected=off
  wires:
  u/1 -> y/1

== system autolibshared/Vehicle Body 3DOF Single Track/Signal Routing/Signal Routing/state2bus/xddot2ax/m^22gn ==
  ay : Inport  Unit=m/s^2
  ax : Inport  Port=2  Unit=m/s^2
  Unit Conversion : UnitConversion
  Unit Conversion1 : UnitConversion
  ay_g : Outport  Unit=gn  VectorParamsAs1DForOutWhenUnconnected=off
  ax_g : Outport  Port=2  Unit=gn  VectorParamsAs1DForOutWhenUnconnected=off
  wires:
  ay/1 -> Unit Conversion/1
  ax/1 -> Unit Conversion1/1
  Unit Conversion/1 -> ay_g/1
  Unit Conversion1/1 -> ax_g/1

== matlab function autolibshared/Vehicle Body 3DOF Single Track/Signal Routing/Signal Routing Dual/state2bus/COMB2I ==
  data: x input size=4; y output size=2
function y = fcn(x)%#codegen
coder.allowpcode('plain')
y = automlvehb2i(x);

== matlab function autolibshared/Vehicle Body 3DOF Single Track/Signal Routing/Signal Routing/state2bus/COMB2I ==
  data: x input size=4; y output size=2
function y = fcn(x)%#codegen
coder.allowpcode('plain')
y = automlvehb2i(x);

== matlab function autolibshared/Vehicle Body 3DOF Single Track/vehicle model ==
  data: delta_f input; delta_r input; mu input; a parameter; b parameter; h parameter; d parameter; w parameter; m parameter; NF parameter; NR parameter; Izz parameter; g parameter; Fxtire_sat parameter size=1; Fytire_sat parameter size=1; trackMode parameter; inputMode parameter; xdot_tol parameter; Fznom parameter size=1; F_f input; F_r input; F_ext input size=3; M_ext input size=3; Cy_f input; Cy_r input; yOut output size=3; FBody output size=3; MBody output size=3; FOut output; FTire output; Fg output size=3; wheelInfo output; stateDer output size=4; stateVec input size=4; status output size=1
function [yOut,FBody,MBody,FOut,FTire,Fg,wheelInfo,stateDer,status] = fcn(delta_f,delta_r,mu,a,b,h,d,w,m,NF,NR,Izz,g,Fxtire_sat,Fytire_sat,trackMode,inputMode,xdot_tol,Fznom,F_f,F_r,F_ext,M_ext,Cy_f,Cy_r,stateVec)%#codegen
coder.allowpcode('plain')
switch trackMode
    case 1
       [yOut,FBody,MBody,FOut,FTire,Fg,wheelInfo,stateDer,status] = automlvehdynbicycle(delta_f,delta_r,mu,a,b,h,m,NF,NR,Izz,g,Fxtire_sat,Fytire_sat,inputMode,xdot_tol,Fznom,F_f,F_r,F_ext,M_ext,Cy_f,Cy_r,stateVec);
    case 2
       [yOut,FBody,MBody,FOut,FTire,Fg,wheelInfo,stateDer,status] = automlvehdyndualtrack(delta_f,delta_r,mu,a,b,h,d,w,m,NF,NR,Izz,g,Fxtire_sat,Fytire_sat,inputMode,xdot_tol,Fznom,F_f,F_r,F_ext,M_ext,Cy_f,Cy_r,stateVec);
end
end

== matlab function autolibshared/Longitudinal Wheel/Wheel Module/Brakes/Drum Brake/Drum Brake/Drum Brake Torque Calculation ==
  data: P input; Ba input; T output; mu input; a input; c input; r input; theta1 input; theta2 input
function T=CalcDrumShoeTorque(P,Ba,mu,a,c,r,theta1,theta2)

   %Convert angles from deg to rad
   theta1=theta1*pi/180.;
   theta2=theta2*pi/180.;
     
   %Calculate torque terms
   sigma=cos(theta2)-cos(theta1);
   
   Numerator=pi*mu*c*r*sigma*Ba^2;
   
   Denominator1=2*mu*(-2*r*sigma-a*(cos(theta1)^2-cos(theta2)^2));

   Denominator2=a*(2*theta1-2*theta2-sin(2*theta1)+sin(2*theta2));
    
   %Right shoe torque
   Tr=P*Numerator/(Denominator1+Denominator2);
   
   %Left shoe torque
   Tl=P*Numerator/(-Denominator1+Denominator2);

   T=Tr+Tl;
   
end

== matlab function autolibshared/Longitudinal Wheel/Longitudinal Basic Magic Tire/Simple Magic Tire ==
  data: ReNom input; Fz input; Fx output size=size(Fz); Omega input; Vx input; MagicPeak input; MagicFxo input; kappaFx input; FzFx input; FxMap input; RollRes input; FZMIN parameter; FZMAX parameter; VXLOW parameter; kappamax parameter; VxMy input; FzMy input; MyMap input; rho input; MagicVert input; My output size=size(Fz); Kappa output size=size(Fz); Re output; FxType input; rollingType input; vertType input; FzTire output
function [Fx,My,Kappa,Re,FzTire] = simpletire(ReNom,Fz,Omega,Vx,...
    MagicPeak,MagicFxo,kappaFx,FzFx,FxMap,RollRes,FZMIN,FZMAX,VXLOW,kappamax,VxMy,FzMy,MyMap,rho,MagicVert,FxType,rollingType,vertType)%#codegen
coder.allowpcode('plain')

switch vertType
    case 0 
        FzTire = Fz;
        Re = ReNom;
    case 1
        [Re,FzTire] = automltireFzmagic(rho,Omega,MagicVert(1),MagicVert(2),MagicVert(3),MagicVert(4),0,0,0,0,0,0,0,...
                                        0,0,0,0,0,0,0,0,0);
    case 2  
        Re = ReNom;
        FzTire = Fz;
    otherwise
        Re = ReNom;
        FzTire = Fz;        
end
Kappa = automltirekappa(ReNom,Omega,Vx,VXLOW,kappamax); 
switch FxType
    case 0
       [Fx] = automltirelongFx(Kappa,Fz,MagicPeak(1),MagicPeak(2),MagicPeak(3),MagicPeak(4),MagicPeak(5),FZMIN,FZMAX);
    case 2
       zeta = [1;1]; 
       Fx = automltirepurelongFx(Kappa,Vx,Fz,MagicFxo(1),MagicFxo(2),...
                                      MagicFxo(3),FZMIN,FZMAX,...
                                      MagicFxo(4),MagicFxo(5),MagicFxo(6),MagicFxo(7),...
                                      MagicFxo(8),MagicFxo(9),MagicFxo(10),MagicFxo(11),...
                                      MagicFxo(12),MagicFxo(13),MagicFxo(14),MagicFxo(15),...
                                      MagicFxo(16),MagicFxo(17),MagicFxo(18),...
                                      MagicFxo(19),MagicFxo(20),...
                                      MagicFxo(21),MagicFxo(22),...
                                      MagicFxo(23),MagicFxo(24),MagicFxo(25),MagicFxo(26),...
                                      MagicFxo(27),MagicFxo(28),MagicFxo(29),MagicFxo(30),...
                                      MagicFxo(31),MagicFxo(32),MagicFxo(33),MagicFxo(34),...
                                      zeta);
    case 3
       [Fx] = automltirelongFxMapped(Kappa,Fz,kappaFx,FzFx,FxMap,FZMIN,FZMAX,MagicPeak(5));
    otherwise
        Fx = zeros(size(Fz));
        Kappa = zeros(size(Fz));
end

switch rollingType
    case 0 %'None'
        My = zeros(size(Fz));
    case 1 %'Simple'
        My = automltirelongMySAE(Fz,Omega,Vx,RollRes(1),RollRes(4),RollRes(5),...
             RollRes(6),RollRes(10),RollRes(11),Re,FZMIN,FZMAX,RollRes(15),RollRes(16));
    case 2 %'Magic Formula'
        My = automltirelongMy(Fx,Fz,Omega,Vx,RollRes(1),RollRes(2), RollRes(3),RollRes(4),RollRes(5),...
            RollRes(6),RollRes(7),RollRes(8),RollRes(9),RollRes(10),RollRes(11),RollRes(12),RollRes(13),RollRes(14),FZMAX,RollRes(15), RollRes(16));
    case 3 %'Mapped Torque'
        My = -automltirelongMyMapped(Omega,Fz,Vx,VxMy,FzMy,MyMap,FZMAX);
    case 4 %'ISO'
        My = automltirelongMyISO(Fz,Omega,RollRes(1),RollRes(4),RollRes(5),...
             RollRes(6),RollRes(7),Re,FZMIN,FZMAX,RollRes(15),RollRes(16));
    otherwise
        My = zeros(size(Fz));
end
end

== stateflow chart autolibshared/Longitudinal Wheel/Wheel Module/Clutch ==
  settings: updateMethod=CONTINUOUS
  state yn = detectSlip(Tout,Tfmaxs) [function]
  state Slipping
  state yn = detectLockup(Tout,Tfmaxs) [function]
  state Locked
  (default) -> Slipping : {Slipping.omegaWheel = 0;}
  Slipping -> Locked : [detectLockup(Tout, Tfmaxs) && (abs(Omega)<=OmegaTol)]
  Locked -> Slipping : [detectSlip(Tout,Tfmaxs)]
      | {
      | Slipping.omegaWheel = 0;
      | }
  data: yn function_output; Tout function_input; Tfmaxs function_input; sf_internal_action_state_placeholder_data local double size=1 =0; omegaWheel local; yn function_output; Tout function_input; Tfmaxs function_input; sf_internal_action_state_placeholder_data local double size=1 =0; Tout input double; Tfmaxs input double; Tfmaxk input double; Omega output double; Omegadot output double; Myb output double; ReactionTorque output double; omegao parameter double; OmegaTol parameter
